simulink model "DF002A_Swp"  (R2013b)
settings: Solver=FixedStepDiscrete  StartTime=0  StopTime=350  FixedStep=ARCHGLBPRM_2MILLISEC_SEC_F32  RelTol=1e-3
undefined symbols (not defined in the file): ARCHGLBPRM_2MILLISEC_SEC_F32, ARCHGLBPRM_2PI_ULS_F32, SwpCfg, SwpDwellTi, SwpFrqList, SwpGain, SwpModEna, SwpOffs, SwpSinAmp, SWPTIUNITCNVN, SwpTranTi, SwpVehSpdChkEna, SwpVehSpdMax
libraries: simulink x6, NexteerUtilities x2
(part 1 of 2)
settings Model: SimulationMode=rapid-accelerator  Creator=hz69by  LastModifiedBy=HZ69BY
settings DataIOCC: SignalLoggingSaveFormat=ModelDataLogs  SaveOutput=off  SignalLogging=off  SaveTime=off
settings OptimizationCC: ExpressionDepthLimit=2147483647
settings DebuggingCC: CheckSSInitialOutputMsg=off  FcnCallInpInsideContextMsg=UseLocalSettings  StateNameClashWarn=warning
settings GRTTargetCC: CombineOutputUpdateFcns=off  GRTInterface=on

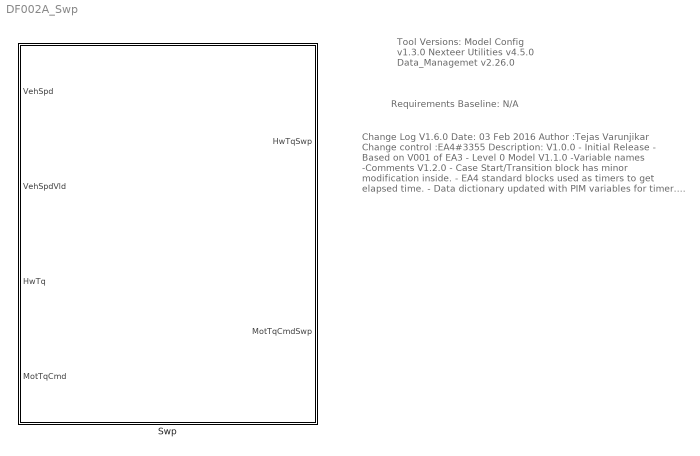
== system DF002A_Swp ==
  note: Requirements Baseline: N/A
  note: Tool Versions:
      |
      | Model Config v1.3.0
      | Nexteer Utilities v4.5.0
      | Data_Managemet v2.26.0
  note: Change Log
      | V1.6.0
      | Date: 03 Feb 2016
      | Author :Tejas Varunjikar
      | Change control :EA4#3355
      |
      | Description:
      | V1.0.0
      | - Initial Release
      | - Based on V001 of EA3
      | - Level 0 Model
      |
      | V1.1.0
      | -Variable names
      | -Comments
      |
      | V1.2.0
      | - Case Start/Transition block has minor modification inside.
      | - EA4 standard blocks used as timers to get elapsed time.
      | - Data dictionary updated with PIM variables for timer. dSwpSwtSt name updated.
      |
      | V1.3.0
      | - Changed switch-case logic placement
      | - Added data store blocks to handle multiple variables
      |
      | V1.4.0
      | - Deleted un-necessary requirements links present in the model
      | - Missing constant SWPTIUNITCNVN added back
      | - Other minor changes
      |
      | V1.5.0
      | - SwpSinAmp made "User Manipulated Variable" in data dictionary
      | - 2nd output name changed to "MotTqCmdSwp" from "MotTqSwp" to match
      | latest NexteerAvailable Signals (EA4) list.
      |
      | V1.6.0
      | - No change in model
      | - Change in data dictionary for SWPENA variable
  Swp : Subsystem

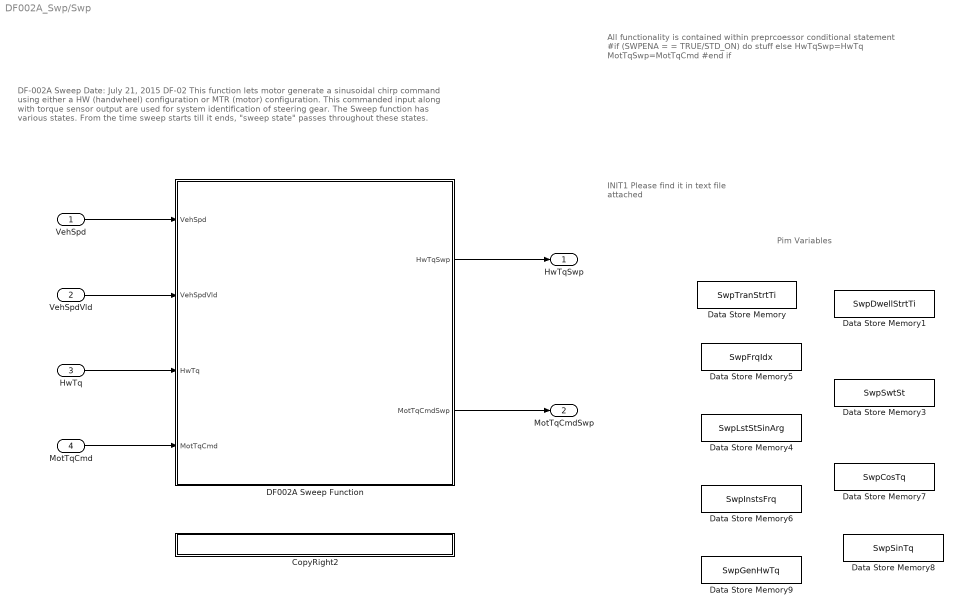
== system DF002A_Swp/Swp ==
  note: Pim Variables
  note: All functionality is contained within preprcoessor conditional statement
      | #if (SWPENA = = TRUE/STD_ON)
      | do stuff
      | else
      | HwTqSwp=HwTq
      | MotTqSwp=MotTqCmd
      | #end if
  note: INIT1
      | Please find it in text file attached
  note: DF-002A  Sweep                                    																 Date: July 21, 2015
      |
      |
      | DF-02
      | This function lets motor generate a sinusoidal chirp command using either a HW (handwheel) configuration or MTR (motor)
      | configuration. This commanded input along with torque sensor output are used for system identification of steering gear.
      |
      | The Sweep function has various states. From the time sweep starts till it ends, "sweep state" passes throughout these states.
  VehSpd : Inport
  VehSpdVld : Inport  Port=2
  HwTq : Inport  Port=3
  MotTqCmd : Inport  Port=4
  CopyRight2 : Subsystem  Description=|  mask(Copyright Information){none=on}
      | Copyright info block.                                               
      |                                                                     
      | Place copyright information at the top of every subsystem in design.
      mask prompts: none "No parameters"
      mask help: Place copyright information at the top of every subsystem in design.
      mask Display:
      | NxtrConf = 'Nexteer Confidential';
      | 
      | sys = bdroot; %handle for the current model ("system")
      | first = get_param(sys,'Created');
      | first = first(end-3:end);  %year is last four digits
      | 
      | last = get_param(sys,'LastModifiedDate');
      | if isempty(last)
      |     last = datestr(now,'yyyy');
      | else
      |     last = last(end-3:end);
      | end
      | 
      | if strcmp(first,last)
      |     fprintf('%s -- Copyright %s Nexteer',NxtrConf,first)
      | else
      |     fprintf('%s -- %s%s- %s Nexteer',NxtrConf,char(169),first,last)
      | end
  DF002A Sweep Function : Subsystem
  Data Store Memory : DataStoreMemory  DataStoreName=SwpTranStrtTi  ReadBeforeWriteMsg=warning  WriteAfterWriteMsg=warning  WriteAfterReadMsg=warning
  Data Store Memory1 : DataStoreMemory  DataStoreName=SwpDwellStrtTi  ReadBeforeWriteMsg=warning  WriteAfterWriteMsg=warning  WriteAfterReadMsg=warning
  Data Store Memory3 : DataStoreMemory  DataStoreName=SwpSwtSt  ReadBeforeWriteMsg=warning  WriteAfterWriteMsg=warning  WriteAfterReadMsg=warning
  Data Store Memory4 : DataStoreMemory  DataStoreName=SwpLstStSinArg  ReadBeforeWriteMsg=warning  WriteAfterWriteMsg=warning  WriteAfterReadMsg=warning
  Data Store Memory5 : DataStoreMemory  DataStoreName=SwpFrqIdx  ReadBeforeWriteMsg=warning  WriteAfterWriteMsg=warning  WriteAfterReadMsg=warning  InitialValue=1
  Data Store Memory6 : DataStoreMemory  DataStoreName=SwpInstsFrq  ReadBeforeWriteMsg=warning  WriteAfterWriteMsg=warning  WriteAfterReadMsg=warning
  Data Store Memory7 : DataStoreMemory  DataStoreName=SwpCosTq  ReadBeforeWriteMsg=warning  WriteAfterWriteMsg=warning  WriteAfterReadMsg=warning
  Data Store Memory8 : DataStoreMemory  DataStoreName=SwpSinTq  ReadBeforeWriteMsg=warning  WriteAfterWriteMsg=warning  WriteAfterReadMsg=warning
  Data Store Memory9 : DataStoreMemory  DataStoreName=SwpGenHwTq  ReadBeforeWriteMsg=warning  WriteAfterWriteMsg=warning  WriteAfterReadMsg=warning
  HwTqSwp : Outport
  MotTqCmdSwp : Outport  Port=2
  wires:
  VehSpd/1 -> DF002A Sweep Function/1(VehSpd)
  VehSpdVld/1 -> DF002A Sweep Function/2(VehSpdVld)
  HwTq/1 -> DF002A Sweep Function/3("HwTq ")
  MotTqCmd/1 -> DF002A Sweep Function/4(MotTqCmd)
  DF002A Sweep Function/1(HwTqSwp) -> HwTqSwp/1
  DF002A Sweep Function/2("MotTqCmdSwp ") -> MotTqCmdSwp/1

== system DF002A_Swp/Swp/CopyRight2 ==

== system DF002A_Swp/Swp/DF002A Sweep Function ==
  VehSpd : Inport
  VehSpdVld : Inport  Port=2
  "HwTq " : Inport  Port=3
  MotTqCmd : Inport  Port=4
  " SwpPer1" : Subsystem
  SwpPer2 : Subsystem
  Zero-Order Hold{1..2,5..6} (4 alike) : ZeroOrderHold  SampleTime=ARCHGLBPRM_2MILLISEC_SEC_F32
  HwTqSwp : Outport
  "MotTqCmdSwp " : Outport  Port=2
  wires:
  " SwpPer1"/2(Sine Torque) -> [SwpSinTq]
  " SwpPer1"/1(OutputHwTrq) -> HwTqSwp/1
  VehSpd/1 -> Zero-Order Hold1/1
  VehSpdVld/1 -> Zero-Order Hold2/1
  "HwTq "/1 -> Zero-Order Hold5/1
  SwpPer2/1(OutputMtrTrq) -> "MotTqCmdSwp "/1
  MotTqCmd/1 -> Zero-Order Hold6/1
  [SwpSinTq] -> SwpPer2/1(SweepTorque)
  Zero-Order Hold1/1 -> " SwpPer1"/1(VehSpd)
  Zero-Order Hold2/1 -> " SwpPer1"/2(VehSpdVld)
  Zero-Order Hold5/1 -> " SwpPer1"/3(InputHwTrq)
  Zero-Order Hold6/1 -> SwpPer2/2(InputMtrTrq)

== system DF002A_Swp/Swp/DF002A Sweep Function/ SwpPer1 ==
  note: This constant defined as a
      | PIM in data dictionary
  note: This constant defined as a
      | PIM in data dictionary
  note: This part of the code generates the sinusoidal sweep signal , and
      | also handles logic associated with the sweep process.
      |
      | This is done regardless of the SweepConfig (HW or MTR). SweepConfig just decides
      |  where to pass the SweepTorque signal calculated. MTR (1) config is default.
      |
      | Once the GenHwTrq is TRUE (1) and VehSpd conditions are satisfied, algorithm
      | transitions between various Sweep State cases (0 to 5), to carry out sweep process.
      |
      | It typically takes more than 320 seconds for whole sweep process to get complete.
      | After sweep is completed, GenHwTrq is defaulted back to 0 (inactive mode).
  VehSpd : Inport
  VehSpdVld : Inport  Port=2
  InputHwTrq : Inport  Port=3
  Check GenHwTrq and VehSpd : Subsystem
  Constant4 : Constant  Value=SwpModEna
  Constant5 : Constant  Value=SwpCfg
  Final Output : Subsystem
  S1 : DataStoreRead  DataStoreName=SwpSinTq
  S3 : DataStoreRead  DataStoreName=SwpSinTq
  S5 : DataStoreRead  DataStoreName=SwpGenHwTq
  Static_Limit : NexteerUtilities/Static_Limit  uprlim=SWPHWTQHILIM  lwrlim=SWPHWTQLOLIM
      settings: AttributesFormatString=|
      | Upper Limit:%<uprlim>
      | Lower Limit:%<lwrlim>
  OutputHwTrq : Outport
  Sine Torque : Outport  Port=2
  wires:
  Final Output/1(OutputHwTrq_HwNm) -> Static_Limit/1  "OutputHwTrq_HwNm"
  S3/1 -> Sine Torque/1
  Constant4/1 -> Final Output/1(SweepModeEn_Cnt)
  Constant5/1 -> Final Output/2(SweepConfig_Cnt)
  S1/1 -> Final Output/3(SweepTorque_HwNm)
  InputHwTrq/1 -> Final Output/4(InputHwTrq_HwNm)
  S5/1 -> Check GenHwTrq and VehSpd/1(GenHwTrq)
  VehSpdVld/1 -> Check GenHwTrq and VehSpd/3(VehSpdValid)  "VehSpdVld"
  VehSpd/1 -> Check GenHwTrq and VehSpd/2(VehSpd_kph)  "VehSpd"
  Static_Limit/1 -> OutputHwTrq/1

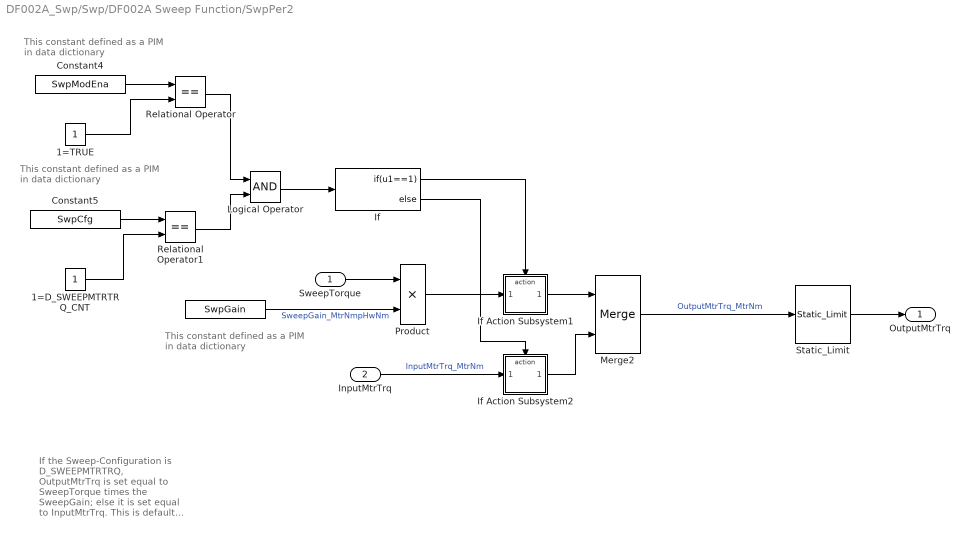
== system DF002A_Swp/Swp/DF002A Sweep Function/SwpPer2 ==
  note: This constant defined as a
      | PIM in data dictionary
  note: If the Sweep-Configuration is D_SWEEPMTRTRQ, OutputMtrTrq is set
      | equal to SweepTorque times the SweepGain; else it is set equal to InputMtrTrq.
      | This is default case.
  note: This constant defined as a
      | PIM in data dictionary
  note: This constant defined as a
      | PIM in data dictionary
  SweepTorque : Inport
  InputMtrTrq : Inport  Port=2
  " " : Constant  Value=SwpGain
  1=D_SWEEPMTRTRQ_CNT : Constant
  1=TRUE : Constant
  Constant4 : Constant  Value=SwpModEna
  Constant5 : Constant  Value=SwpCfg
  If : If  IfExpression=u1==1
  If Action Subsystem1 : Subsystem  TreatAsAtomicUnit=on  mask(pass thru, version Nov 30, 2012){nIn=1}
      mask prompts: nIn "Number of input signals"
      mask help:
      | This block passes its input straight through without modification.
      |
      | Enter the number of signals to pass through (integer 1 to 5).
      mask Callback nIn:
      | thisBlock = gcb;
      | a = get_param(thisBlock,'MaskValues');
      | b = cell2mat(a);
      | c = str2num(b);
      | 
      | if c<1 c=1; end
      | if c>5 c=5; end
      | 
      | for idx=1:c
      |     sIdx = num2str(idx);
      |     oldblock = [thisBlock '/In' sIdx];
      |     if strcmp(get_param(oldblock,'BlockType'),'Ground')
      |          newblock = 'built-in/Inport';
      |         pos = get_param(oldblock,'Position');
      |         orient = get_param(oldblock,'Orientation');
      |         delete_block(oldblock);
      |         add_block(newblock,oldblock,'Position',pos, 'Orientation',orient);
      |     end
      | 
      |     oldblock = [thisBlock '/Out' sIdx];
      |     if strcmp(get_param(oldblock,'BlockType'),'Terminator')
      |         newblock = 'built-in/Outport';
      |         pos = get_param(oldblock,'Position');
      |         orient = get_param(oldblock,'Orientation');
      |         delete_block(oldblock);
      |         add_block(newblock,oldblock,'Position',pos, 'Orientation',orient);
      |     end
      | end
      | 
      | for idx=c+1:5
      |     sIdx = num2str(idx);
      |     oldblock = [thisBlock '/In' sIdx];
      |     if strcmp(get_param(oldblock,'BlockType'),'Inport')
      |         newblock = 'built-in/Ground';
      |         pos = get_param(oldblock,'Position');
      |         orient = get_param(oldblock,'Orientation');
      |         delete_block(oldblock);
      |         add_block(newblock,oldblock,'Position',pos, 'Orientation',orient);
      |     end
      | 
      |     oldblock = [thisBlock '/Out' sIdx];
      |     if strcmp(get_param(oldblock,'BlockType'),'Outport')
      |         newblock = 'built-in/Terminator';
      |         pos = get_param(oldblock,'Position');
      |         orient = get_param(oldblock,'Orientation');
      |         delete_block(oldblock);
      |         add_block(newblock,oldblock,'Position',pos, 'Orientation',orient);
      |     end
      | end
      | 
      | 
      | 
      | clear thisBlock oldblock newblock orient pos a b c idx sIdx ;
      mask Display: fprintf('pass\nthru')
  If Action Subsystem2 : Subsystem  TreatAsAtomicUnit=on  mask(pass thru, version Nov 30, 2012){nIn=1}
      mask prompts: nIn "Number of input signals"
      mask help:
      | This block passes its input straight through without modification.
      |
      | Enter the number of signals to pass through (integer 1 to 5).
      mask Callback nIn:
      | thisBlock = gcb;
      | a = get_param(thisBlock,'MaskValues');
      | b = cell2mat(a);
      | c = str2num(b);
      | 
      | if c<1 c=1; end
      | if c>5 c=5; end
      | 
      | for idx=1:c
      |     sIdx = num2str(idx);
      |     oldblock = [thisBlock '/In' sIdx];
      |     if strcmp(get_param(oldblock,'BlockType'),'Ground')
      |          newblock = 'built-in/Inport';
      |         pos = get_param(oldblock,'Position');
      |         orient = get_param(oldblock,'Orientation');
      |         delete_block(oldblock);
      |         add_block(newblock,oldblock,'Position',pos, 'Orientation',orient);
      |     end
      | 
      |     oldblock = [thisBlock '/Out' sIdx];
      |     if strcmp(get_param(oldblock,'BlockType'),'Terminator')
      |         newblock = 'built-in/Outport';
      |         pos = get_param(oldblock,'Position');
      |         orient = get_param(oldblock,'Orientation');
      |         delete_block(oldblock);
      |         add_block(newblock,oldblock,'Position',pos, 'Orientation',orient);
      |     end
      | end
      | 
      | for idx=c+1:5
      |     sIdx = num2str(idx);
      |     oldblock = [thisBlock '/In' sIdx];
      |     if strcmp(get_param(oldblock,'BlockType'),'Inport')
      |         newblock = 'built-in/Ground';
      |         pos = get_param(oldblock,'Position');
      |         orient = get_param(oldblock,'Orientation');
      |         delete_block(oldblock);
      |         add_block(newblock,oldblock,'Position',pos, 'Orientation',orient);
      |     end
      | 
      |     oldblock = [thisBlock '/Out' sIdx];
      |     if strcmp(get_param(oldblock,'BlockType'),'Outport')
      |         newblock = 'built-in/Terminator';
      |         pos = get_param(oldblock,'Position');
      |         orient = get_param(oldblock,'Orientation');
      |         delete_block(oldblock);
      |         add_block(newblock,oldblock,'Position',pos, 'Orientation',orient);
      |     end
      | end
      | 
      | 
      | 
      | clear thisBlock oldblock newblock orient pos a b c idx sIdx ;
      mask Display: fprintf('pass\nthru')
  Logical Operator : Logic  AllPortsSameDT=off  OutDataTypeStr=boolean
  Merge2 : Merge  InitialOutput=0
  Product : Product  RndMeth=Zero
  Relational Operator : RelationalOperator  Operator===  OutDataTypeStr=boolean
  Relational Operator1 : RelationalOperator  Operator===  OutDataTypeStr=boolean
  Static_Limit : NexteerUtilities/Static_Limit  uprlim=SYSGLBPRM_MOTTQCMDHILIM_MOTNWTMTR_F32  lwrlim=SYSGLBPRM_MOTTQCMDLOLIM_MOTNWTMTR_F32
      settings: AttributesFormatString=|
      | Upper Limit:%<uprlim>
      | Lower Limit:%<lwrlim>
  OutputMtrTrq : Outport
  wires:
  InputMtrTrq/1 -> If Action Subsystem2/1(In1)  "InputMtrTrq_MtrNm"
  Constant5/1 -> Relational Operator1/1
  SweepTorque/1 -> Product/1
  Constant4/1 -> Relational Operator/1
  Merge2/1 -> Static_Limit/1  "OutputMtrTrq_MtrNm"
  If Action Subsystem2/1(Out1) -> Merge2/2
  If Action Subsystem1/1(Out1) -> Merge2/1
  If/2 -> If Action Subsystem2/Action
  If/1 -> If Action Subsystem1/Action
  Logical Operator/1 -> If/1
  Relational Operator1/1 -> Logical Operator/2
  Relational Operator/1 -> Logical Operator/1
  1=D_SWEEPMTRTRQ_CNT/1 -> Relational Operator1/2
  1=TRUE/1 -> Relational Operator/2
  Product/1 -> If Action Subsystem1/1(In1)
  " "/1 -> Product/2  "SweepGain_MtrNmpHwNm"
  Static_Limit/1 -> OutputMtrTrq/1

== system DF002A_Swp/Swp/DF002A Sweep Function/ SwpPer1/Check GenHwTrq and VehSpd ==
  note: When GenHwTrq=TRUE and Vehicle Speed Criteria is satisfied,
      | all inputs are just passed through (and reset timer is not activated).
      |
      | When GenHwTrq=FALSE, everything is reset to default.
      |
      | If Vehicle speed criteria is not satisfied during GenHwTrq=TRUE,
      | sweep process goes to RAMP state and exits.
  GenHwTrq : Inport
  VehSpd_kph : Inport  Port=2
  VehSpdValid : Inport  Port=3
  If : If  IfExpression=u1==1
  "If GenHwTrq=FALSE, Reset all variables to Default." : Subsystem  TreatAsAtomicUnit=on
  "If GenHwTrq=TRUE, Check Vehicle Speed Criteria" : Subsystem  TreatAsAtomicUnit=on
  wires:
  GenHwTrq/1 -> If/1
  VehSpd_kph/1 -> "If GenHwTrq=TRUE, Check Vehicle Speed Criteria"/1(VehSpd_Kph)
  VehSpdValid/1 -> "If GenHwTrq=TRUE, Check Vehicle Speed Criteria"/2(VehSpdValid)
  If/1 -> "If GenHwTrq=TRUE, Check Vehicle Speed Criteria"/Action
  If/2 -> "If GenHwTrq=FALSE, Reset all variables to Default."/Action

== system DF002A_Swp/Swp/DF002A Sweep Function/ SwpPer1/Final Output ==
  note: If the Sweep-Configuration is D_SWEEPHWTRQ, OutputHwTrq is set
      | equal to SweepTorque; else it is set equal to InputHwTrq.
  SweepModeEn_Cnt : Inport
  SweepConfig_Cnt : Inport  Port=2
  SweepTorque_HwNm : Inport  Port=3
  InputHwTrq_HwNm : Inport  Port=4
  1=TRUE : Constant
  2=D_SWEEPHWTRQ_CNT : Constant  Value=2
  If : If  IfExpression=u1==1
  If Action Subsystem1 : Subsystem  TreatAsAtomicUnit=on  mask(pass thru, version Nov 30, 2012){nIn=1}
      mask prompts: nIn "Number of input signals"
      mask help:
      | This block passes its input straight through without modification.
      |
      | Enter the number of signals to pass through (integer 1 to 5).
      mask Callback nIn:
      | thisBlock = gcb;
      | a = get_param(thisBlock,'MaskValues');
      | b = cell2mat(a);
      | c = str2num(b);
      | 
      | if c<1 c=1; end
      | if c>5 c=5; end
      | 
      | for idx=1:c
      |     sIdx = num2str(idx);
      |     oldblock = [thisBlock '/In' sIdx];
      |     if strcmp(get_param(oldblock,'BlockType'),'Ground')
      |          newblock = 'built-in/Inport';
      |         pos = get_param(oldblock,'Position');
      |         orient = get_param(oldblock,'Orientation');
      |         delete_block(oldblock);
      |         add_block(newblock,oldblock,'Position',pos, 'Orientation',orient);
      |     end
      | 
      |     oldblock = [thisBlock '/Out' sIdx];
      |     if strcmp(get_param(oldblock,'BlockType'),'Terminator')
      |         newblock = 'built-in/Outport';
      |         pos = get_param(oldblock,'Position');
      |         orient = get_param(oldblock,'Orientation');
      |         delete_block(oldblock);
      |         add_block(newblock,oldblock,'Position',pos, 'Orientation',orient);
      |     end
      | end
      | 
      | for idx=c+1:5
      |     sIdx = num2str(idx);
      |     oldblock = [thisBlock '/In' sIdx];
      |     if strcmp(get_param(oldblock,'BlockType'),'Inport')
      |         newblock = 'built-in/Ground';
      |         pos = get_param(oldblock,'Position');
      |         orient = get_param(oldblock,'Orientation');
      |         delete_block(oldblock);
      |         add_block(newblock,oldblock,'Position',pos, 'Orientation',orient);
      |     end
      | 
      |     oldblock = [thisBlock '/Out' sIdx];
      |     if strcmp(get_param(oldblock,'BlockType'),'Outport')
      |         newblock = 'built-in/Terminator';
      |         pos = get_param(oldblock,'Position');
      |         orient = get_param(oldblock,'Orientation');
      |         delete_block(oldblock);
      |         add_block(newblock,oldblock,'Position',pos, 'Orientation',orient);
      |     end
      | end
      | 
      | 
      | 
      | clear thisBlock oldblock newblock orient pos a b c idx sIdx ;
      mask Display: fprintf('pass\nthru')
  If Action Subsystem2 : Subsystem  TreatAsAtomicUnit=on  mask(pass thru, version Nov 30, 2012){nIn=1}
      mask prompts: nIn "Number of input signals"
      mask help:
      | This block passes its input straight through without modification.
      |
      | Enter the number of signals to pass through (integer 1 to 5).
      mask Callback nIn:
      | thisBlock = gcb;
      | a = get_param(thisBlock,'MaskValues');
      | b = cell2mat(a);
      | c = str2num(b);
      | 
      | if c<1 c=1; end
      | if c>5 c=5; end
      | 
      | for idx=1:c
      |     sIdx = num2str(idx);
      |     oldblock = [thisBlock '/In' sIdx];
      |     if strcmp(get_param(oldblock,'BlockType'),'Ground')
      |          newblock = 'built-in/Inport';
      |         pos = get_param(oldblock,'Position');
      |         orient = get_param(oldblock,'Orientation');
      |         delete_block(oldblock);
      |         add_block(newblock,oldblock,'Position',pos, 'Orientation',orient);
      |     end
      | 
      |     oldblock = [thisBlock '/Out' sIdx];
      |     if strcmp(get_param(oldblock,'BlockType'),'Terminator')
      |         newblock = 'built-in/Outport';
      |         pos = get_param(oldblock,'Position');
      |         orient = get_param(oldblock,'Orientation');
      |         delete_block(oldblock);
      |         add_block(newblock,oldblock,'Position',pos, 'Orientation',orient);
      |     end
      | end
      | 
      | for idx=c+1:5
      |     sIdx = num2str(idx);
      |     oldblock = [thisBlock '/In' sIdx];
      |     if strcmp(get_param(oldblock,'BlockType'),'Inport')
      |         newblock = 'built-in/Ground';
      |         pos = get_param(oldblock,'Position');
      |         orient = get_param(oldblock,'Orientation');
      |         delete_block(oldblock);
      |         add_block(newblock,oldblock,'Position',pos, 'Orientation',orient);
      |     end
      | 
      |     oldblock = [thisBlock '/Out' sIdx];
      |     if strcmp(get_param(oldblock,'BlockType'),'Outport')
      |         newblock = 'built-in/Terminator';
      |         pos = get_param(oldblock,'Position');
      |         orient = get_param(oldblock,'Orientation');
      |         delete_block(oldblock);
      |         add_block(newblock,oldblock,'Position',pos, 'Orientation',orient);
      |     end
      | end
      | 
      | 
      | 
      | clear thisBlock oldblock newblock orient pos a b c idx sIdx ;
      mask Display: fprintf('pass\nthru')
  Logical Operator : Logic  AllPortsSameDT=off  OutDataTypeStr=boolean
  Merge2 : Merge  InitialOutput=0
  Relational Operator : RelationalOperator  Operator===  OutDataTypeStr=boolean
  Relational Operator1 : RelationalOperator  Operator===  OutDataTypeStr=boolean
  OutputHwTrq_HwNm : Outport
  wires:
  1=TRUE/1 -> Relational Operator/2
  2=D_SWEEPHWTRQ_CNT/1 -> Relational Operator1/2
  Relational Operator/1 -> Logical Operator/1
  Relational Operator1/1 -> Logical Operator/2
  Logical Operator/1 -> If/1
  If/1 -> If Action Subsystem2/Action
  If/2 -> If Action Subsystem1/Action
  If Action Subsystem2/1(Out1) -> Merge2/1
  If Action Subsystem1/1(Out1) -> Merge2/2
  Merge2/1 -> OutputHwTrq_HwNm/1
  SweepModeEn_Cnt/1 -> Relational Operator/1
  SweepTorque_HwNm/1 -> If Action Subsystem2/1(In1)
  SweepConfig_Cnt/1 -> Relational Operator1/1
  InputHwTrq_HwNm/1 -> If Action Subsystem1/1(In1)

== system DF002A_Swp/Swp/DF002A Sweep Function/SwpPer2/If Action Subsystem1 ==
  note: Do not modify these blocks manually.  They
      | are generated programatically.  Changing the
      | number of blocks available or their names requires
      | corresponding changes to Callback and Initialization
      | routines.
      |
      | Do not change the "Display" tab of mask editor.  The
      | outport names are created programatically in the
      | "Initialize" section.
  note: Change Log:
      | Oct 12, 2012  Created by Kevin Derry as a 1-input, 1-output block
      | Nov 30, 2012  dynamically configurable for 1 to 5 ports.
  In1 : Inport
  Action Port : ActionPort  ActionType=then
  In{2..5} (4 alike) : Ground
  Out{2..5} (4 alike) : Terminator
  Out1 : Outport
  wires:
  In5/1 -> Out5/1
  In4/1 -> Out4/1
  In3/1 -> Out3/1
  In2/1 -> Out2/1
  In1/1 -> Out1/1

== system DF002A_Swp/Swp/DF002A Sweep Function/SwpPer2/If Action Subsystem2 ==
  note: Change Log:
      | Oct 12, 2012  Created by Kevin Derry as a 1-input, 1-output block
      | Nov 30, 2012  dynamically configurable for 1 to 5 ports.
  note: Do not modify these blocks manually.  They
      | are generated programatically.  Changing the
      | number of blocks available or their names requires
      | corresponding changes to Callback and Initialization
      | routines.
      |
      | Do not change the "Display" tab of mask editor.  The
      | outport names are created programatically in the
      | "Initialize" section.
  In1 : Inport
  Action Port : ActionPort  ActionType=else
  In{2..5} (4 alike) : Ground
  Out{2..5} (4 alike) : Terminator
  Out1 : Outport
  wires:
  In1/1 -> Out1/1
  In2/1 -> Out2/1
  In3/1 -> Out3/1
  In4/1 -> Out4/1
  In5/1 -> Out5/1

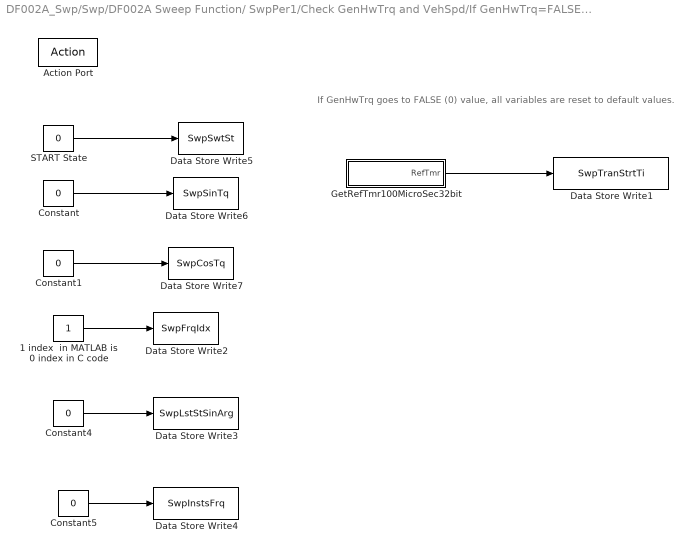
== system DF002A_Swp/Swp/DF002A Sweep Function/ SwpPer1/Check GenHwTrq and VehSpd/If GenHwTrq=FALSE, Reset all variables to Default. ==
  note: If GenHwTrq goes to FALSE (0) value, all variables are reset to default values.
  Action Port : ActionPort  ActionType=else
  1 index  in MATLAB is 0 index in C code : Constant
  Constant{,1,4..5} (4 alike) : Constant  Value=0
  Data Store Write1 : DataStoreWrite  RequirementInfo={} %GIDa_76ea2039_3667_4286_9bdb_9e1b482b3599  DataStoreName=SwpTranStrtTi
  Data Store Write2 : DataStoreWrite  RequirementInfo={} %GIDa_75a91380_f945_4669_b6ab_cea7d2a6fada  DataStoreName=SwpFrqIdx
  Data Store Write3 : DataStoreWrite  RequirementInfo={} %GIDa_c391bfba_452f_4d68_a9f4_0c0bdfe91b7e  DataStoreName=SwpLstStSinArg
  Data Store Write4 : DataStoreWrite  RequirementInfo={} %GIDa_cf6af025_690b_45c2_8828_eaa30f9d7731  DataStoreName=SwpInstsFrq
  Data Store Write5 : DataStoreWrite  RequirementInfo={} %GIDa_1d09d1ba_0a0c_4ceb_836d_84e37ea5dd1e  DataStoreName=SwpSwtSt
  Data Store Write6 : DataStoreWrite  RequirementInfo={} %GIDa_3c2f8b80_44de_49b5_8b04_bc8162702532  DataStoreName=SwpSinTq
  Data Store Write7 : DataStoreWrite  RequirementInfo={} %GIDa_d1ef2b1d_32fc_4e5c_879a_b63b79572f74  DataStoreName=SwpCosTq
  GetRefTmr100MicroSec32bit : Subsystem  RequirementInfo={} %GIDa_319f7b53_9c49_4767_b35b_bb10f84b5412
  START State : Constant  Value=0
  wires:
  START State/1 -> Data Store Write5/1
  Constant/1 -> Data Store Write6/1
  Constant1/1 -> Data Store Write7/1
  1 index  in MATLAB is 0 index in C code/1 -> Data Store Write2/1
  Constant4/1 -> Data Store Write3/1
  Constant5/1 -> Data Store Write4/1
  GetRefTmr100MicroSec32bit/1(RefTmr) -> Data Store Write1/1

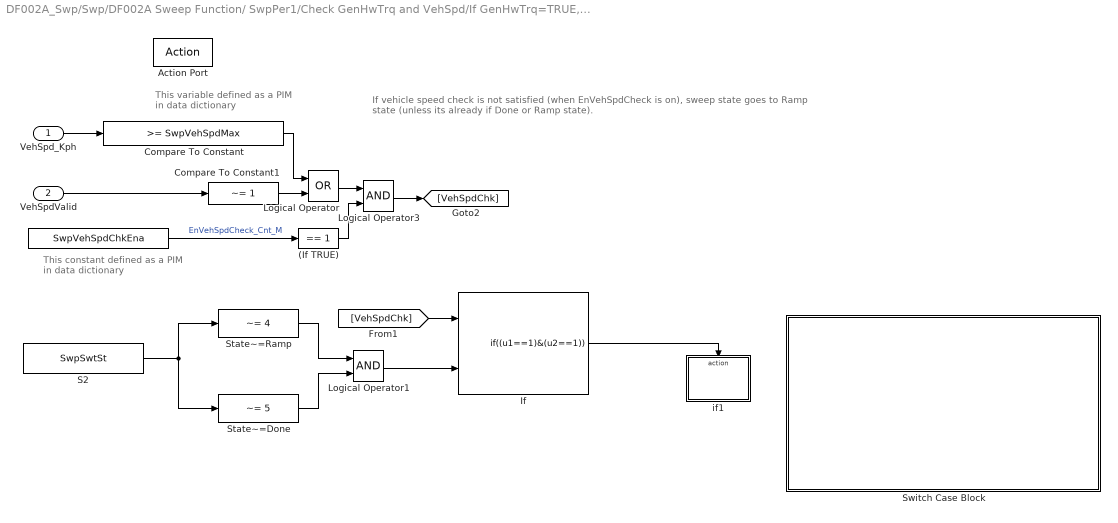
== system DF002A_Swp/Swp/DF002A Sweep Function/ SwpPer1/Check GenHwTrq and VehSpd/If GenHwTrq=TRUE, Check Vehicle Speed Criteria ==
  note: This variable defined as a
      | PIM in data dictionary
  note: If vehicle speed check is not satisfied (when EnVehSpdCheck is on),
      | sweep state goes to Ramp state (unless its already if Done or Ramp state).
  note: This constant defined as a
      | PIM in data dictionary
  VehSpd_Kph : Inport
  VehSpdValid : Inport  Port=2
  Action Port : ActionPort  ActionType=then
  " " : Constant  Value=SwpVehSpdChkEna
  (If TRUE) : simulink/Logic and Bit Operations/Compare To Constant  relop===  const=1  OutDataTypeStr=uint8
  Compare To Constant : simulink/Logic and Bit Operations/Compare To Constant  relop=>=  const=SwpVehSpdMax  OutDataTypeStr=uint8
      settings: AttributesFormatString=%<const>
  Compare To Constant1 : simulink/Logic and Bit Operations/Compare To Constant  relop=~=  const=1  OutDataTypeStr=uint8
  If : If  NumInputs=2  IfExpression=(u1==1)&(u2==1)  ShowElse=off
  Logical Operator : Logic  Operator=OR  AllPortsSameDT=off  OutDataTypeStr=boolean
  Logical Operator1 : Logic  AllPortsSameDT=off  OutDataTypeStr=boolean
  Logical Operator3 : Logic  AllPortsSameDT=off  OutDataTypeStr=boolean
  S2 : DataStoreRead  DataStoreName=SwpSwtSt
  State~=Done : simulink/Logic and Bit Operations/Compare To Constant  relop=~=  const=5  OutDataTypeStr=uint8
  State~=Ramp : simulink/Logic and Bit Operations/Compare To Constant  relop=~=  const=4  OutDataTypeStr=uint8
  Switch Case Block : Subsystem  Priority=1
      settings: AttributesFormatString=Priority=%<Priority>
  if1 : Subsystem  RequirementInfo={} %GIDa_a1992620_0bd1_4e77_921c_ad7961ef1e0e  Priority=0  TreatAsAtomicUnit=on
      settings: AttributesFormatString=Priority=%<Priority>
  wires:
  VehSpd_Kph/1 -> Compare To Constant/1
  Compare To Constant/1 -> Logical Operator/1
  Compare To Constant1/1 -> Logical Operator/2
  VehSpdValid/1 -> Compare To Constant1/1
  S2/1 -> State~=Ramp/1, State~=Done/1
  State~=Ramp/1 -> Logical Operator1/1
  State~=Done/1 -> Logical Operator1/2
  Logical Operator1/1 -> If/2
  If/1 -> if1/Action
  Logical Operator/1 -> Logical Operator3/1
  " "/1 -> (If TRUE)/1  "EnVehSpdCheck_Cnt_M"
  (If TRUE)/1 -> Logical Operator3/2
  Logical Operator3/1 -> [VehSpdChk]
  [VehSpdChk] -> If/1

== system DF002A_Swp/Swp/DF002A Sweep Function/ SwpPer1/Final Output/If Action Subsystem1 ==
  note: Do not modify these blocks manually.  They
      | are generated programatically.  Changing the
      | number of blocks available or their names requires
      | corresponding changes to Callback and Initialization
      | routines.
      |
      | Do not change the "Display" tab of mask editor.  The
      | outport names are created programatically in the
      | "Initialize" section.
  note: Change Log:
      | Oct 12, 2012  Created by Kevin Derry as a 1-input, 1-output block
      | Nov 30, 2012  dynamically configurable for 1 to 5 ports.
  In1 : Inport
  Action Port : ActionPort  ActionType=else
  In{2..5} (4 alike) : Ground
  Out{2..5} (4 alike) : Terminator
  Out1 : Outport
  wires:
  In5/1 -> Out5/1
  In4/1 -> Out4/1
  In3/1 -> Out3/1
  In2/1 -> Out2/1
  In1/1 -> Out1/1

== system DF002A_Swp/Swp/DF002A Sweep Function/ SwpPer1/Final Output/If Action Subsystem2 ==
  note: Do not modify these blocks manually.  They
      | are generated programatically.  Changing the
      | number of blocks available or their names requires
      | corresponding changes to Callback and Initialization
      | routines.
      |
      | Do not change the "Display" tab of mask editor.  The
      | outport names are created programatically in the
      | "Initialize" section.
  note: Change Log:
      | Oct 12, 2012  Created by Kevin Derry as a 1-input, 1-output block
      | Nov 30, 2012  dynamically configurable for 1 to 5 ports.
  In1 : Inport
  Action Port : ActionPort  ActionType=then
  In{2..5} (4 alike) : Ground
  Out{2..5} (4 alike) : Terminator
  Out1 : Outport
  wires:
  In5/1 -> Out5/1
  In4/1 -> Out4/1
  In3/1 -> Out3/1
  In2/1 -> Out2/1
  In1/1 -> Out1/1

== system DF002A_Swp/Swp/DF002A Sweep Function/ SwpPer1/Check GenHwTrq and VehSpd/If GenHwTrq=FALSE, Reset all variables to Default./GetRefTmr100MicroSec32bit ==
  note: 1 count = 100 uSec
  note: seconds
  note: microseconds
  note: counts
  note: Wrap-to-zero
  note: GetRefTmr100MicroSec32bit
  Clock : Clock
  CopyRight2 : Subsystem  Description=|  mask(Copyright Information){none=on}
      | Copyright info block.                                               
      |                                                                     
      | Place copyright information at the top of every subsystem in design.
      mask prompts: none "No parameters"
      mask help: Place copyright information at the top of every subsystem in design.
      mask Display:
      | NxtrConf = 'Nexteer Confidential';
      | 
      | sys = bdroot; %handle for the current model ("system")
      | first = get_param(sys,'Created');
      | if(isempty(first))
      |     first = datestr(now,'yyyy');
      | else
      |     first = first(end-3:end);  %year is last four digits
      | end
      | 
      | last = get_param(sys,'LastModifiedDate');
      | if isempty(last)
      |     last = datestr(now,'yyyy');
      | else
      |     last = last(end-3:end);
      | end
      | 
      | if strcmp(first,last)
      |     fprintf('%s -- Copyright %s Nexteer',NxtrConf,first)
      | else
      |     fprintf('%s -- %s%s- %s Nexteer',NxtrConf,char(169),first,last)
      | end
  Count per uSec : Constant  Value=0.01
  Data Type Conversion1 : DataTypeConversion  OutDataTypeStr=uint32
  Divide1 : Product  Inputs=**
  Divide2 : Product  Inputs=*/
  Max Counts : Constant  Value=2^32-1
  Product1 : Product
  Product2 : Product
  Rounding : Rounding
  Subtract1 : Sum  Inputs=+-
  uSec per Sec : Constant  Value=1000000
  RefTmr : Outport
  wires:
  Product2/1 -> Subtract1/2
  Subtract1/1 -> Data Type Conversion1/1
  Rounding/1 -> Product2/1
  Divide2/1 -> Rounding/1
  Max Counts/1 -> Divide2/2, Product2/2
  Divide1/1 -> Divide2/1, Subtract1/1
  Product1/1 -> Divide1/1
  Clock/1 -> Product1/1
  Count per uSec/1 -> Divide1/2
  uSec per Sec/1 -> Product1/2
  Data Type Conversion1/1 -> RefTmr/1

== system DF002A_Swp/Swp/DF002A Sweep Function/ SwpPer1/Check GenHwTrq and VehSpd/If GenHwTrq=TRUE, Check Vehicle Speed Criteria/Switch Case Block ==
  note: Cases
      | 0:Start, 1: Transition
      | 2:Dwell, 3:Stop
      | 4:Ramp, 5: Done
  Default: Switch Case Action : Subsystem  TreatAsAtomicUnit=on
  Dwell/Stop: Switch Case Action Subsystem1 : Subsystem  TreatAsAtomicUnit=on
  Ramp: Switch Case Action : Subsystem  TreatAsAtomicUnit=on
  S2 : DataStoreRead  DataStoreName=SwpSwtSt
  "Start/Transition: Switch Case Action Subsystem " : Subsystem  TreatAsAtomicUnit=on
  Switch Case : SwitchCase  CaseConditions={[0,1],[2,3],4,5}  ShowDefaultCase=off
  wires:
  Switch Case/1 -> "Start/Transition: Switch Case Action Subsystem "/Action
  Switch Case/2 -> Dwell/Stop: Switch Case Action Subsystem1/Action
  Switch Case/4 -> Default: Switch Case Action/Action
  Switch Case/3 -> Ramp: Switch Case Action/Action
  S2/1 -> Switch Case/1

== system DF002A_Swp/Swp/DF002A Sweep Function/ SwpPer1/Check GenHwTrq and VehSpd/If GenHwTrq=TRUE, Check Vehicle Speed Criteria/if1 ==
  Action Port : ActionPort  ActionType=then
  CopyRight2 : Subsystem  Description=|  mask(Copyright Information){none=on}
      | Copyright info block.                                               
      |                                                                     
      | Place copyright information at the top of every subsystem in design.
      mask prompts: none "No parameters"
      mask help: Place copyright information at the top of every subsystem in design.
      mask Display:
      | NxtrConf = 'Nexteer Confidential';
      | 
      | sys = bdroot; %handle for the current model ("system")
      | first = get_param(sys,'Created');
      | if(isempty(first))
      |     first = datestr(now,'yyyy');
      | else
      |     first = first(end-3:end);  %year is last four digits
      | end
      | 
      | last = get_param(sys,'LastModifiedDate');
      | if isempty(last)
      |     last = datestr(now,'yyyy');
      | else
      |     last = last(end-3:end);
      | end
      | 
      | if strcmp(first,last)
      |     fprintf('%s -- Copyright %s Nexteer',NxtrConf,first)
      | else
      |     fprintf('%s -- %s%s- %s Nexteer',NxtrConf,char(169),first,last)
      | end
  Data Store Write1 : DataStoreWrite  RequirementInfo={} %GIDa_cd8200a6_1e03_43a5_9d36_1a78c66614a7  DataStoreName=SwpTranStrtTi
  Data Store Write2 : DataStoreWrite  RequirementInfo={} %GIDa_39d7e3b9_d795_4c72_992d_3e5bf79c8fa5  DataStoreName=SwpSwtSt
  GetRefTmr100MicroSec32bit : Subsystem  RequirementInfo={} %GIDa_2c6bed81_ddfe_4592_bd86_5b845654c52f
  Ramp State : Constant  Value=4
  wires:
  Ramp State/1 -> Data Store Write2/1
  GetRefTmr100MicroSec32bit/1(RefTmr) -> Data Store Write1/1

== system DF002A_Swp/Swp/DF002A Sweep Function/ SwpPer1/Check GenHwTrq and VehSpd/If GenHwTrq=FALSE, Reset all variables to Default./GetRefTmr100MicroSec32bit/CopyRight2 ==

== system DF002A_Swp/Swp/DF002A Sweep Function/ SwpPer1/Check GenHwTrq and VehSpd/If GenHwTrq=TRUE, Check Vehicle Speed Criteria/Switch Case Block/Default: Switch Case Action ==
  note: Done state indicates that sweep process is done.
      | Various States are reset to default values.
  Action Port : ActionPort  ActionType=case
  CosineSweepTorque : Constant  Value=0
  Data Store Write1 : DataStoreWrite  RequirementInfo={} %GIDa_233844bb_a259_49b6_84c6_4e7b2c521404  DataStoreName=SwpCosTq
  Data Store Write2 : DataStoreWrite  RequirementInfo={} %GIDa_8e2a1ae0_466b_4ca5_bed9_b3737f106abd  DataStoreName=SwpSinTq
  Data Store Write3 : DataStoreWrite  RequirementInfo={} %GIDa_9d23b157_9ed8_4b56_9858_3f2671b15e49  DataStoreName=SwpGenHwTq
  DefaultGenHwTq (False) : Constant  Value=0
  SineSweepTorque : Constant  Value=0
  wires:
  CosineSweepTorque/1 -> Data Store Write1/1
  SineSweepTorque/1 -> Data Store Write2/1
  DefaultGenHwTq (False)/1 -> Data Store Write3/1

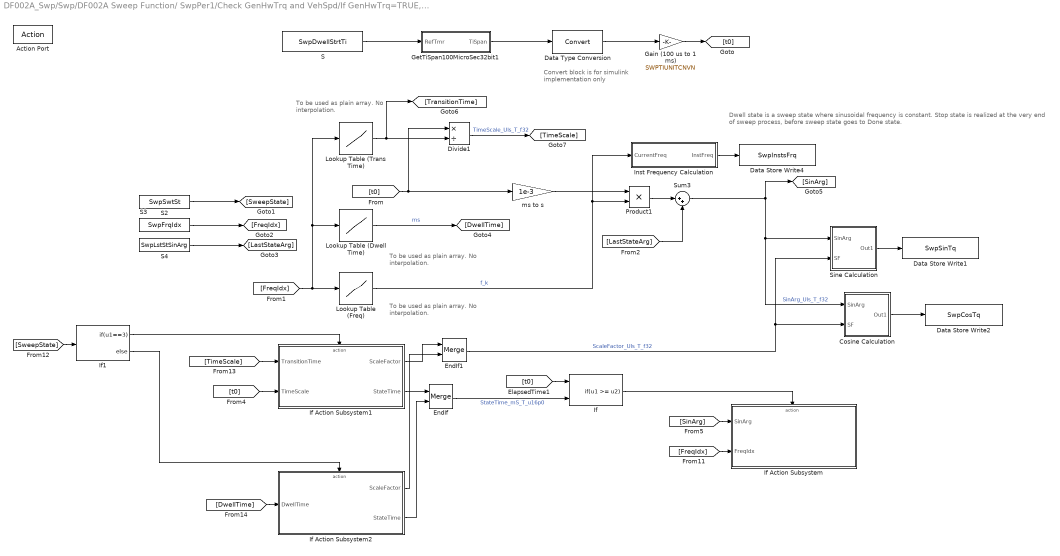
== system DF002A_Swp/Swp/DF002A Sweep Function/ SwpPer1/Check GenHwTrq and VehSpd/If GenHwTrq=TRUE, Check Vehicle Speed Criteria/Switch Case Block/Dwell//Stop: Switch Case Action Subsystem1 ==
  note: To be used as plain array.
      |  No interpolation.
  note: Dwell state is a sweep state where sinusoidal frequency is constant.
      | Stop state is realized at the very end of sweep process, before sweep
      | state goes to Done state.
  note: To be used as plain array.
      |  No interpolation.
  note: To be used as plain array.
      |  No interpolation.
  note: Convert block is for simulink
      | implementation only
  Action Port : ActionPort  ActionType=case
  Cosine Calculation : Subsystem
  Data Store Write1 : DataStoreWrite  RequirementInfo={} %GIDa_4952933d_442d_4d11_885f_9869bfdfe3c0  DataStoreName=SwpSinTq
  Data Store Write2 : DataStoreWrite  RequirementInfo={} %GIDa_ffe7bd7c_4c22_47ff_b203_9f925a53c0b5  DataStoreName=SwpCosTq
  Data Store Write4 : DataStoreWrite  RequirementInfo={} %GIDa_ceaf59c2_c75f_4773_8481_eaad42140ce1  DataStoreName=SwpInstsFrq
  Data Type Conversion : DataTypeConversion
  Divide1 : Product  Inputs=*/
  EndIf : Merge
  EndIf1 : Merge
  Gain (100 us to 1 ms) : Gain  Gain=SWPTIUNITCNVN
      settings: AttributesFormatString=%<Gain>
  GetTiSpan100MicroSec32bit1 : Subsystem  RequirementInfo={} %GIDa_1bf2f083_9634_4b81_a71e_003e76b247c9
  If : If  NumInputs=2  IfExpression=u1 >= u2  ShowElse=off
  If Action Subsystem : Subsystem  TreatAsAtomicUnit=on
  If Action Subsystem1 : Subsystem  TreatAsAtomicUnit=on
  If Action Subsystem2 : Subsystem  TreatAsAtomicUnit=on
  If1 : If  IfExpression=u1==3
  Inst Frequency Calculation : Subsystem
  Lookup Table (Dwell Time) : Lookup  InputValues=1:length(SwpDwellTi)  Table=SwpDwellTi
      settings: AttributesFormatString=%<Table>
  Lookup Table (Freq) : Lookup  InputValues=1:length(SwpFrqList)  Table=SwpFrqList
      settings: AttributesFormatString=%<Table>
  Lookup Table (Trans Time) : Lookup  InputValues=1:length(SwpTranTi)  Table=SwpTranTi
      settings: AttributesFormatString=%<Table>
  Product1 : Product  RndMeth=Zero
  S : DataStoreRead  DataStoreName=SwpDwellStrtTi
  S2 : DataStoreRead  DataStoreName=SwpSwtSt
  S3 : DataStoreRead  DataStoreName=SwpFrqIdx
  S4 : DataStoreRead  DataStoreName=SwpLstStSinArg
  Sine Calculation : Subsystem
  Sum3 : Sum  Inputs=|++
  ms to s : Gain  Gain=1e-3
  wires:
  [FreqIdx] -> Lookup Table (Trans Time)/1, Lookup Table (Dwell Time)/1, Lookup Table (Freq)/1
  Lookup Table (Dwell Time)/1 -> [DwellTime]  "ms"
  Product1/1 -> Sum3/1
  [LastStateArg] -> Sum3/2
  Sine Calculation/1(Out1) -> Data Store Write1/1
  EndIf1/1 -> Sine Calculation/2(SF), Cosine Calculation/2(SF)  "ScaleFactor_Uls_T_f32"
  Sum3/1 -> Sine Calculation/1(SinArg), Cosine Calculation/1(SinArg), [SinArg]  "SinArg_Uls_T_f32"
  Cosine Calculation/1(Out1) -> Data Store Write2/1
  GetTiSpan100MicroSec32bit1/1(TiSpan) -> Data Type Conversion/1
  S2/1 -> [SweepState]
  S3/1 -> [FreqIdx]
  S4/1 -> [LastStateArg]
  ms to s/1 -> Product1/1
  [t0] -> If/1
  [SinArg] -> If Action Subsystem/1(SinArg)
  [FreqIdx] -> If Action Subsystem/2(FreqIdx)
  EndIf/1 -> If/2  "StateTime_mS_T_u16p0"
  Lookup Table (Freq)/1 -> Product1/2, Inst Frequency Calculation/1(CurrentFreq)  "f_k"
  [DwellTime] -> If Action Subsystem2/1(DwellTime)
  [SweepState] -> If1/1
  If Action Subsystem1/2(StateTime) -> EndIf/1
  If/1 -> If Action Subsystem/Action
  Inst Frequency Calculation/1(InstFreq) -> Data Store Write4/1
  S/1 -> GetTiSpan100MicroSec32bit1/1(RefTmr)
  Gain (100 us to 1 ms)/1 -> [t0]
  Data Type Conversion/1 -> Gain (100 us to 1 ms)/1
  If1/1 -> If Action Subsystem1/Action
  [TimeScale] -> If Action Subsystem1/1(TransitionTime)
  If1/2 -> If Action Subsystem2/Action
  [t0] -> If Action Subsystem1/2(TimeScale)
  If Action Subsystem2/2(StateTime) -> EndIf/2
  If Action Subsystem1/1(ScaleFactor) -> EndIf1/1
  If Action Subsystem2/1(ScaleFactor) -> EndIf1/2
  [t0] -> Divide1/1, ms to s/1
  Lookup Table (Trans Time)/1 -> Divide1/2, [TransitionTime]
  Divide1/1 -> [TimeScale]  "TimeScale_Uls_T_f32"

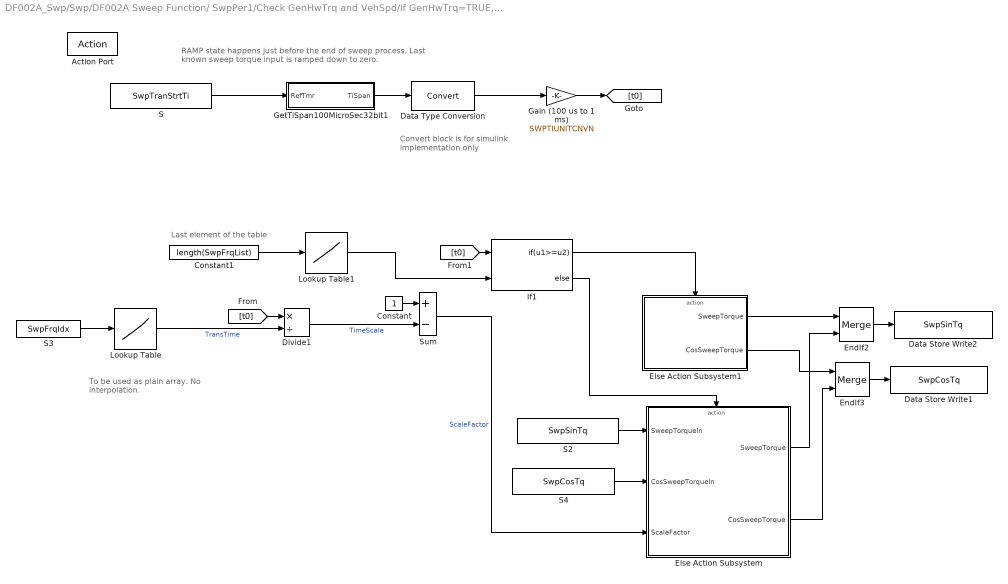
== system DF002A_Swp/Swp/DF002A Sweep Function/ SwpPer1/Check GenHwTrq and VehSpd/If GenHwTrq=TRUE, Check Vehicle Speed Criteria/Switch Case Block/Ramp: Switch Case Action ==
  note: Last element of the table
  note: RAMP state happens just before the end of sweep process.
      | Last known sweep torque input is ramped down to zero.
  note: To be used as plain array.
      |  No interpolation.
  note: Convert block is for simulink
      | implementation only
  Action Port : ActionPort  ActionType=case
  Constant : Constant
  Constant1 : Constant  Value=length(SwpFrqList)
  Data Store Write1 : DataStoreWrite  RequirementInfo={} %GIDa_752dab2b_063e_4551_9740_b05d18e75e9f  DataStoreName=SwpCosTq
  Data Store Write2 : DataStoreWrite  RequirementInfo={} %GIDa_e96efc1c_f791_4fac_a2f2_64a597aee935  DataStoreName=SwpSinTq
  Data Type Conversion : DataTypeConversion
  Divide1 : Product  Inputs=*/
  Else Action Subsystem : Subsystem  TreatAsAtomicUnit=on
  Else Action Subsystem1 : Subsystem  TreatAsAtomicUnit=on
  EndIf2 : Merge  InitialOutput=0
  EndIf3 : Merge  InitialOutput=0
  Gain (100 us to 1 ms) : Gain  Gain=SWPTIUNITCNVN
      settings: AttributesFormatString=%<Gain>
  GetTiSpan100MicroSec32bit1 : Subsystem  RequirementInfo={} %GIDa_09b64144_a998_4dd5_8907_58becf0d6cc8
  If1 : If  NumInputs=2  IfExpression=u1>=u2
  Lookup Table : Lookup  InputValues=1:length(SwpTranTi)  Table=SwpTranTi
      settings: AttributesFormatString=%<Table>
  Lookup Table1 : Lookup  InputValues=1:length(SwpTranTi)  Table=SwpTranTi
      settings: AttributesFormatString=%<Table>
  S : DataStoreRead  DataStoreName=SwpTranStrtTi
  S2 : DataStoreRead  DataStoreName=SwpSinTq
  S3 : DataStoreRead  DataStoreName=SwpFrqIdx
  S4 : DataStoreRead  DataStoreName=SwpCosTq
  Sum : Sum  Inputs=+-
  wires:
  Lookup Table/1 -> Divide1/2  "TransTime"
  [t0] -> Divide1/1
  S3/1 -> Lookup Table/1
  [t0] -> If1/1
  Else Action Subsystem1/1(SweepTorque) -> EndIf2/1
  Else Action Subsystem/1(SweepTorque) -> EndIf2/2
  Else Action Subsystem1/2(CosSweepTorque) -> EndIf3/1
  Else Action Subsystem/2(CosSweepTorque) -> EndIf3/2
  EndIf2/1 -> Data Store Write2/1
  EndIf3/1 -> Data Store Write1/1
  If1/2 -> Else Action Subsystem/Action
  Sum/1 -> Else Action Subsystem/3(ScaleFactor)  "ScaleFactor"
  S2/1 -> Else Action Subsystem/1(SweepTorqueIn)
  S4/1 -> Else Action Subsystem/2(CosSweepTorqueIn)
  If1/1 -> Else Action Subsystem1/Action
  Constant/1 -> Sum/1
  Divide1/1 -> Sum/2  "TimeScale"
  S/1 -> GetTiSpan100MicroSec32bit1/1(RefTmr)
  Gain (100 us to 1 ms)/1 -> [t0]
  Data Type Conversion/1 -> Gain (100 us to 1 ms)/1
  Constant1/1 -> Lookup Table1/1
  Lookup Table1/1 -> If1/2
  GetTiSpan100MicroSec32bit1/1(TiSpan) -> Data Type Conversion/1

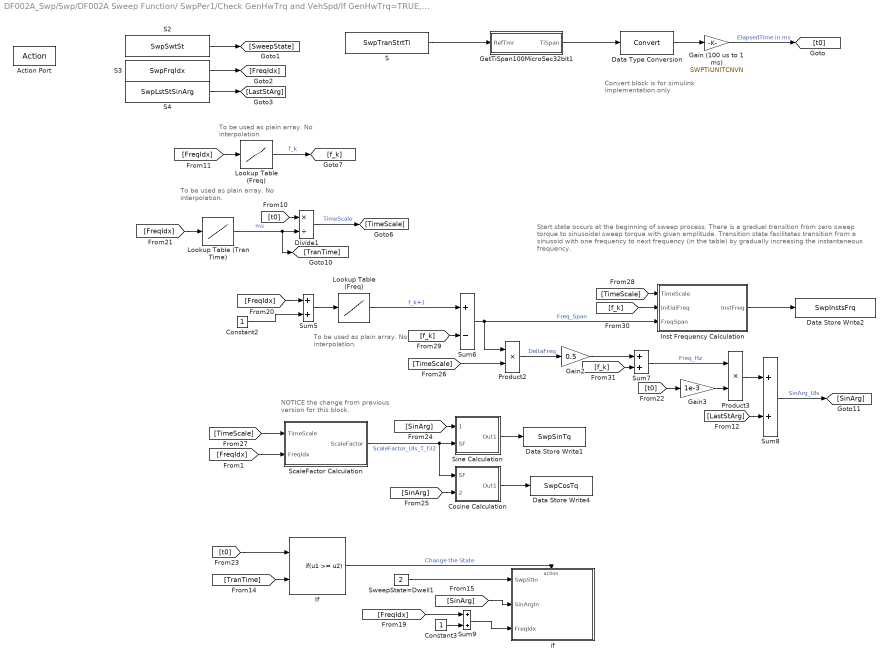
== system DF002A_Swp/Swp/DF002A Sweep Function/ SwpPer1/Check GenHwTrq and VehSpd/If GenHwTrq=TRUE, Check Vehicle Speed Criteria/Switch Case Block/Start//Transition: Switch Case Action Subsystem  ==
  note: NOTICE the change from previous
      |  version for this block.
  note: Convert block is for simulink
      | implementation only
  note: To be used as plain array.
      |  No interpolation.
  note: To be used as plain array.
      |  No interpolation.
  note: Start state occurs at the beginning of sweep process. There is a gradual
      | transition from zero sweep torque to sinusoidal sweep torque with given amplitude.
      |
      | Transition state facilitates transition from a sinusoid with one frequency to next
      | frequency (in the table) by gradually increasing the instantaneous frequency.
  note: To be used as plain array.
      |  No interpolation.
  Action Port : ActionPort  ActionType=case
  Constant2 : Constant
  Constant3 : Constant
  Cosine Calculation : Subsystem
  Data Store Write1 : DataStoreWrite  RequirementInfo={} %GIDa_4e741c16_c069_44dc_9e6e_42565a5c0fdc  DataStoreName=SwpSinTq
  Data Store Write2 : DataStoreWrite  RequirementInfo={} %GIDa_d762cac5_7551_40bc_ade8_1bcf46ae1863  DataStoreName=SwpInstsFrq
  Data Store Write4 : DataStoreWrite  RequirementInfo={} %GIDa_e0507c2d_4b8d_4565_a790_6a29c68b6583  DataStoreName=SwpCosTq
  Data Type Conversion : DataTypeConversion
  Divide1 : Product  Inputs=*/
  Gain (100 us to 1 ms) : Gain  Gain=SWPTIUNITCNVN
      settings: AttributesFormatString=%<Gain>
  Gain2 : Gain  Gain=0.5
  Gain3 : Gain  Gain=1e-3
  GetTiSpan100MicroSec32bit1 : Subsystem  RequirementInfo={} %GIDa_34597255_2ead_4ca2_8c2a_756ecb09755d
  If : If  NumInputs=2  IfExpression=u1 >= u2  ShowElse=off
  Inst Frequency Calculation : Subsystem
  Lookup Table (Freq) : Lookup  InputValues=1:length(SwpFrqList)  Table=SwpFrqList
      settings: AttributesFormatString=%<Table>
  "Lookup Table (Freq) " : Lookup  InputValues=1:length(SwpFrqList)  Table=SwpFrqList
      settings: AttributesFormatString=%<Table>
  Lookup Table (Tran Time) : Lookup  InputValues=1:length(SwpTranTi)  Table=SwpTranTi
      settings: AttributesFormatString=%<Table>
  Product2 : Product  RndMeth=Zero
  Product3 : Product  RndMeth=Zero
  S : DataStoreRead  DataStoreName=SwpTranStrtTi
  S2 : DataStoreRead  DataStoreName=SwpSwtSt
  S3 : DataStoreRead  DataStoreName=SwpFrqIdx
  S4 : DataStoreRead  DataStoreName=SwpLstStSinArg
  ScaleFactor Calculation : Subsystem
  Sine Calculation : Subsystem
  Sum{5,7..9} (4 alike) : Sum
  Sum6 : Sum  Inputs=+-
  SweepState=Dwell1 : Constant  Value=2
  if : Subsystem  RequirementInfo={} %GIDa_79fed533_33aa_4152_ab6d_024ebc7e602b  TreatAsAtomicUnit=on
  wires:
  Sine Calculation/1(Out1) -> Data Store Write1/1
  Cosine Calculation/1(Out1) -> Data Store Write4/1
  S2/1 -> [SweepState]
  S3/1 -> [FreqIdx]
  S4/1 -> [LastStArg]
  [FreqIdx] -> "Lookup Table (Freq) "/1
  Constant2/1 -> Sum5/2
  Sum5/1 -> Lookup Table (Freq)/1
  [t0] -> Divide1/1
  Lookup Table (Tran Time)/1 -> Divide1/2, [TranTime]  "ms"
  Product2/1 -> Gain2/1  "DeltaFreq"
  Product3/1 -> Sum8/1
  [LastStArg] -> Sum8/2
  Sum8/1 -> [SinArg]  "SinArg_Uls"
  [t0] -> If/1
  [TranTime] -> If/2
  If/1 -> if/Action  "Change the State"
  Constant3/1 -> Sum9/2
  SweepState=Dwell1/1 -> if/1(SwpStIn)
  [SinArg] -> if/2(SinArgIn)
  [FreqIdx] -> Sum9/1
  Sum9/1 -> if/3(FreqIdx)
  Inst Frequency Calculation/1(InstFreq) -> Data Store Write2/1
  [FreqIdx] -> Sum5/1
  [FreqIdx] -> Lookup Table (Tran Time)/1
  [t0] -> Gain3/1
  Lookup Table (Freq)/1 -> Sum6/1  "f_k+1"
  [SinArg] -> Sine Calculation/1(SinArg)
  [SinArg] -> Cosine Calculation/2(SinArg)
  Divide1/1 -> [TimeScale]  "TimeScale"
  [TimeScale] -> Inst Frequency Calculation/1(TimeScale)
  "Lookup Table (Freq) "/1 -> [f_k]  "f_k"
  [f_k] -> Sum6/2
  [f_k] -> Inst Frequency Calculation/2(InitialFreq)
  Gain3/1 -> Product3/2
  Gain2/1 -> Sum7/1
  [f_k] -> Sum7/2
  Sum7/1 -> Product3/1  "Freq_Hz"
  [TimeScale] -> ScaleFactor Calculation/1(TimeScale)
  [FreqIdx] -> ScaleFactor Calculation/2(FreqIdx)
  ScaleFactor Calculation/1(ScaleFactor) -> Sine Calculation/2(SF), Cosine Calculation/1(SF)  "ScaleFactor_Uls_T_f32"
  [TimeScale] -> Product2/2
  Sum6/1 -> Inst Frequency Calculation/3(FreqSpan), Product2/1  "Freq_Span"
  S/1 -> GetTiSpan100MicroSec32bit1/1(RefTmr)
  GetTiSpan100MicroSec32bit1/1(TiSpan) -> Data Type Conversion/1
  Gain (100 us to 1 ms)/1 -> [t0]  "ElapsedTime in ms"
  Data Type Conversion/1 -> Gain (100 us to 1 ms)/1

== system DF002A_Swp/Swp/DF002A Sweep Function/ SwpPer1/Check GenHwTrq and VehSpd/If GenHwTrq=TRUE, Check Vehicle Speed Criteria/if1/CopyRight2 ==

== system DF002A_Swp/Swp/DF002A Sweep Function/ SwpPer1/Check GenHwTrq and VehSpd/If GenHwTrq=TRUE, Check Vehicle Speed Criteria/if1/GetRefTmr100MicroSec32bit ==
  note: 1 count = 100 uSec
  note: seconds
  note: microseconds
  note: counts
  note: Wrap-to-zero
  note: GetRefTmr100MicroSec32bit
  Clock : Clock
  CopyRight2 : Subsystem  Description=|  mask(Copyright Information){none=on}
      | Copyright info block.                                               
      |                                                                     
      | Place copyright information at the top of every subsystem in design.
      mask prompts: none "No parameters"
      mask help: Place copyright information at the top of every subsystem in design.
      mask Display:
      | NxtrConf = 'Nexteer Confidential';
      | 
      | sys = bdroot; %handle for the current model ("system")
      | first = get_param(sys,'Created');
      | if(isempty(first))
      |     first = datestr(now,'yyyy');
      | else
      |     first = first(end-3:end);  %year is last four digits
      | end
      | 
      | last = get_param(sys,'LastModifiedDate');
      | if isempty(last)
      |     last = datestr(now,'yyyy');
      | else
      |     last = last(end-3:end);
      | end
      | 
      | if strcmp(first,last)
      |     fprintf('%s -- Copyright %s Nexteer',NxtrConf,first)
      | else
      |     fprintf('%s -- %s%s- %s Nexteer',NxtrConf,char(169),first,last)
      | end
  Count per uSec : Constant  Value=0.01
  Data Type Conversion1 : DataTypeConversion  OutDataTypeStr=uint32
  Divide1 : Product  Inputs=**
  Divide2 : Product  Inputs=*/
  Max Counts : Constant  Value=2^32-1
  Product1 : Product
  Product2 : Product
  Rounding : Rounding
  Subtract1 : Sum  Inputs=+-
  uSec per Sec : Constant  Value=1000000
  RefTmr : Outport
  wires:
  Product2/1 -> Subtract1/2
  Subtract1/1 -> Data Type Conversion1/1
  Rounding/1 -> Product2/1
  Divide2/1 -> Rounding/1
  Max Counts/1 -> Divide2/2, Product2/2
  Divide1/1 -> Divide2/1, Subtract1/1
  Product1/1 -> Divide1/1
  Clock/1 -> Product1/1
  Count per uSec/1 -> Divide1/2
  uSec per Sec/1 -> Product1/2
  Data Type Conversion1/1 -> RefTmr/1
